simulink model "halfCarModel"  (Simulink 8.8)
settings: Solver=FixedStepAuto  StartTime=0.0  StopTime=5  FixedStep=.005  RelTol=1e-3
settings Model: SuppressorTable=22 serialization::archive 11 0 3 0 0 0 0 0  Creator=Devon  LastModifiedBy=Devon
settings DataIOCC: LimitDataPoints=off  SaveFormat=Dataset  SignalLoggingSaveFormat=Dataset
settings OptimizationCC: LifeSpan=auto
settings DebuggingCC: UnderspecifiedInitializationDetection=Simplified  MergeDetectMultiDrivingBlocksExec=error  FcnCallInpInsideContextMsg=error  StateNameClashWarn=none  SFUnexpectedBacktrackingDiag=error  SFNoUnconditionalDefaultTransitionDiag=error  SFExecutionAtInitializationDiag=warning
settings HardwareCC: ProdBitPerPointer=64  ProdBitPerSizeT=64  ProdBitPerPtrDiffT=64  ProdLargestAtomicFloat=Float  ProdIntDivRoundTo=Zero  ProdEndianess=LittleEndian  ProdWordSize=64  ProdHWDeviceType=Intel->x86-64 (Windows64)
settings ModelReferenceCC: PropagateSignalLabelsOutOfModel=on
settings GRTTargetCC: TargetLangStandard=C99 (ISO)  GeneratePreprocessorConditionals=Use local settings  CombineOutputUpdateFcns=on  GRTInterface=off
settings ConfigComp: CovMetricSettings=dwe  CovHtmlReporting=off  CovSaveCumulativeToWorkspaceVar=off  CovSaveSingleToWorkspaceVar=off  CovExternalEMLEnable=on

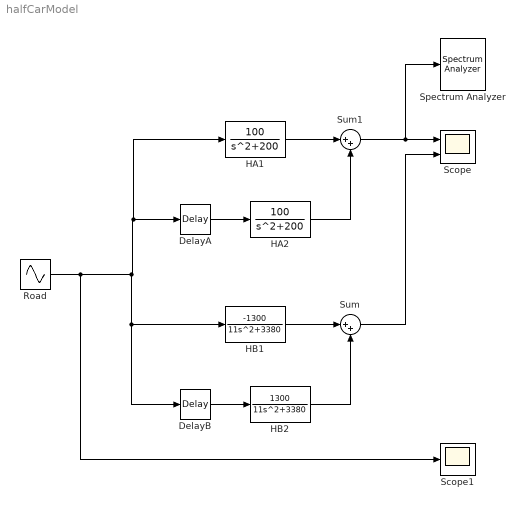
== system halfCarModel ==
  DelayA : TransportDelay  DelayTime=0.117117117117117
  DelayB : TransportDelay  DelayTime=0.117117117117117
  HA1 : TransferFcn  Numerator=100  Denominator=[1 0 200]
  HA2 : TransferFcn  Numerator=100  Denominator=[1 0 200]
  HB1 : TransferFcn  Numerator=-1300  Denominator=[11 0 3380]
  HB2 : TransferFcn  Numerator=1300  Denominator=[11 0 3380]
  Road : Sin  Amplitude=0.015  Frequency=69.7433569096934  SampleTime=0
  Scope : Scope  NumInputPorts=2
  Scope1 : Scope
  Spectrum Analyzer : SpectrumAnalyzer
  Sum : Sum  Inputs=|++
  Sum1 : Sum  Inputs=|++
  wires:
  Road/1 -> Scope1/1, HB1/1, DelayB/1, HA1/1, DelayA/1
  Sum1/1 -> Spectrum Analyzer/1, Scope/1
  Sum/1 -> Scope/2
  HA1/1 -> Sum1/1
  DelayA/1 -> HA2/1
  HA2/1 -> Sum1/2
  HB1/1 -> Sum/1
  HB2/1 -> Sum/2
  DelayB/1 -> HB2/1
